simulink model "decentralized_closedloop"  (Simulink 7.4)
settings: Solver=ode45  StartTime=0.0  StopTime=400  FixedStep=0.05  MaxStep=0.05  RelTol=1e-3
values from neighbouring files (symbols this model uses):
  Ts = 0.05    [test_predictions.m]
  UWT = kron(eye(m),diag(UW'))    [test_predictions.m]
  xtotalsize = xsize + 2*sum(n_delay) + 2*dsize    [MpcSetup.m]
  yref = 0.2    [test_predictions.m]
  YWT = kron(eye(p),diag(YW'))    [test_predictions.m]
undefined symbols (not defined in the file or in its folder): n_controller_iterations, ucontrolsize, yss
libraries: lib_parallel_comp x1
settings Model: Creator=chkajon  LastModifiedBy=katie
settings SFSimCC: SimUserSources=../call_qpoases_m/call_qpoases.c
settings SFSimCC: SimUserIncludeDirs=|
  | ../call_qpoases_m/qpoases3/src
  | ../call_qpoases_m/qpoases3/include

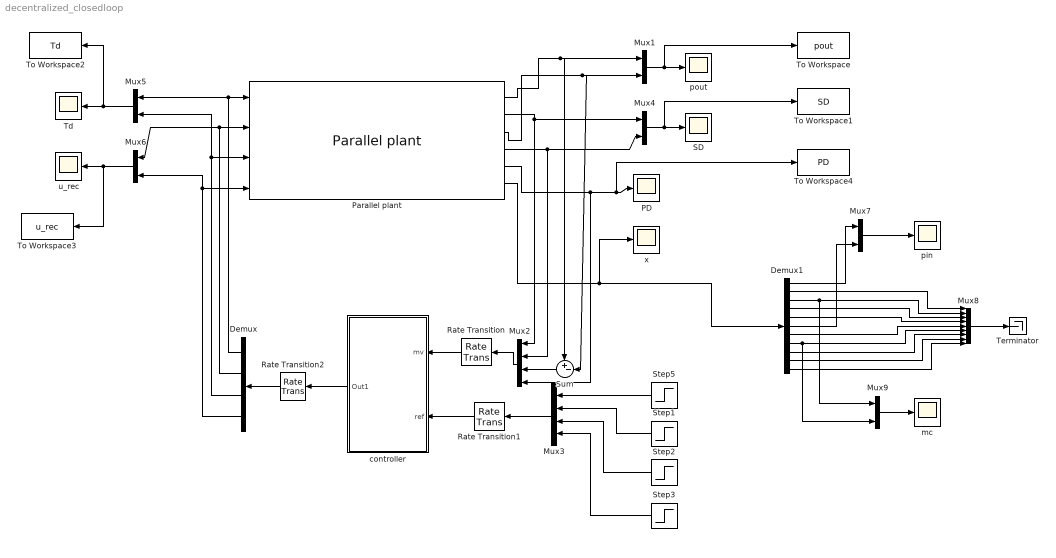
== system decentralized_closedloop ==
  Demux : Demux
  Demux1 : Demux  Outputs=11
  Mux{1,4..7,9} (6 alike) : Mux  Inputs=2
  Mux2 : Mux
  Mux3 : Mux
  Mux8 : Mux  Inputs=9
  PD : Scope
      settings: TimeRange=100  YMin=1.1  YMax=1.26  SaveName=SD1  DataFormat=Array
  Parallel plant : lib_parallel_comp/Parallel plant  SystemSampleTime=-1  disturbances_on=on  disturbances_symm=off  dist_t_in=tdist  dist1_in=udist1  dist2_in=udist2
  Rate Transition : RateTransition  X0=yss
  Rate Transition1 : RateTransition  X0=yref
  Rate Transition2 : RateTransition
  SD : Scope
      settings: TimeRange=100  YMin=-2.5  YMax=1.5  SaveName=SD3  DataFormat=Array
  Step1 : Step  Time=0  Before=0.22  After=0.22  SampleTime=0
  Step2 : Step  Time=0  After=0  SampleTime=0
  Step3 : Step  Time=0  Before=1.12  After=1.12  SampleTime=0
  Step5 : Step  Time=0  Before=0.22  After=0.22  SampleTime=0
  Sum : Sum  Inputs=+-|  OutDataType=fixdt(1, 16)  OutScaling=2^0
  Td : Scope
      settings: TimeRange=100  YMin=-0.15  YMax=0.25  SaveName=SD4  DataFormat=Array
  Terminator : Terminator
  To Workspace : ToWorkspace  VariableName=pout  SampleTime=-1  SaveFormat=Structure With Time
  To Workspace1 : ToWorkspace  VariableName=SD  SampleTime=-1  SaveFormat=Structure With Time
  To Workspace2 : ToWorkspace  VariableName=Td  SampleTime=-1  SaveFormat=Structure With Time
  To Workspace3 : ToWorkspace  VariableName=u_rec  SampleTime=-1  SaveFormat=Structure With Time
  To Workspace4 : ToWorkspace  VariableName=PD  SampleTime=-1  SaveFormat=Structure With Time
  controller : Subsystem  TreatAsAtomicUnit=on  SystemSampleTime=Ts
  mc : Scope
      settings: TimeRange=200  YMin=0.1175  YMax=0.155  SaveName=SD8  DataFormat=Array
  pin : Scope
      settings: TimeRange=200  YMin=0.89  YMax=1  SaveName=SD7  DataFormat=Array
  pout : Scope
      settings: TimeRange=100  YMin=1.38778e-017  YMax=0.4  SaveName=SD2  DataFormat=Array
  u_rec : Scope
      settings: TimeRange=100  YMin=-3.46945e-018  YMax=0.11  SaveName=SD5  DataFormat=Array
  x : Scope
      settings: TimeRange=85  YMin=1.1125  YMax=1.1141  SaveName=SD6  DataFormat=Array
  wires:
  controller/1(Out1) -> Rate Transition2/1
  Mux2/1 -> Rate Transition/1
  Mux3/1 -> Rate Transition1/1
  Rate Transition/1 -> controller/1(mv)
  Rate Transition1/1 -> controller/2(ref)
  Rate Transition2/1 -> Demux/1
  Demux/1 -> Mux5/1, Parallel plant/1
  Demux/2 -> Mux6/1, Parallel plant/2
  Demux/3 -> Mux5/2, Parallel plant/3
  Demux/4 -> Mux6/2, Parallel plant/4
  Step5/1 -> Mux3/1
  Step1/1 -> Mux3/2
  Step2/1 -> Mux3/3
  Step3/1 -> Mux3/4
  Parallel plant/1 -> Mux1/1, Sum/1
  Parallel plant/5 -> PD/1, To Workspace4/1, Mux2/4
  Parallel plant/2 -> Mux4/1, Mux2/1
  Parallel plant/3 -> Mux1/2, Sum/2
  Mux4/1 -> SD/1, To Workspace1/1
  Mux1/1 -> pout/1, To Workspace/1
  Mux5/1 -> Td/1, To Workspace2/1
  Mux6/1 -> u_rec/1, To Workspace3/1
  Parallel plant/6 -> x/1, Demux1/1
  Demux1/1 -> Mux7/1
  Demux1/6 -> Mux7/2
  Demux1/2 -> Mux8/1
  Demux1/3 -> Mux8/2, Mux9/1
  Demux1/4 -> Mux8/3
  Demux1/5 -> Mux8/4
  Demux1/7 -> Mux8/5
  Demux1/8 -> Mux8/6, Mux9/2
  Demux1/9 -> Mux8/7
  Demux1/10 -> Mux8/8
  Demux1/11 -> Mux8/9
  Mux8/1 -> Terminator/1
  Mux7/1 -> pin/1
  Mux9/1 -> mc/1
  Parallel plant/4 -> Mux4/2, Mux2/2
  Sum/1 -> Mux2/3

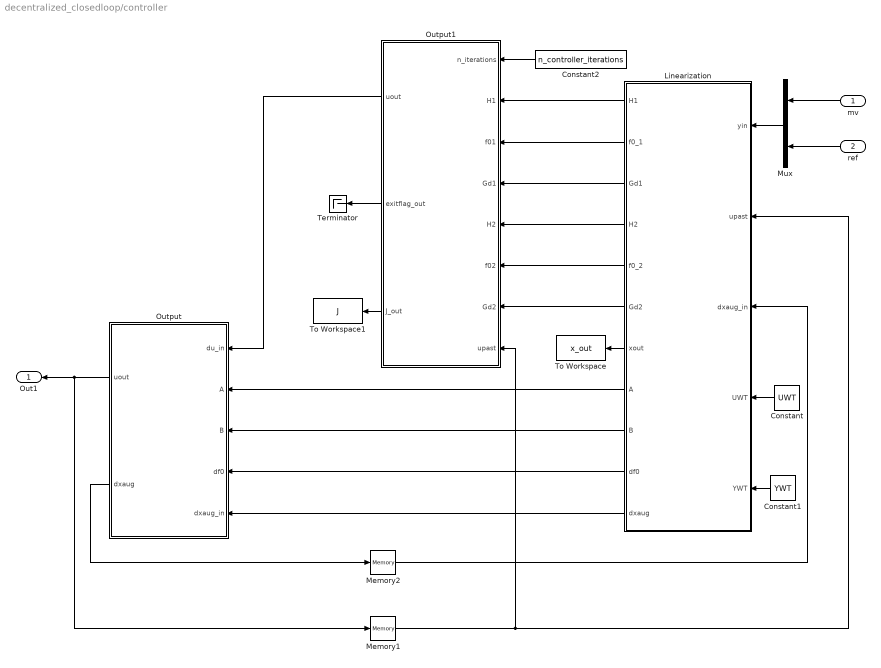
== system decentralized_closedloop/controller ==
  mv : Inport
  ref : Inport  Port=2
  Constant : Constant  Value=UWT  OutDataType=fixdt(1, 16)  OutScaling=2^0
  Constant1 : Constant  Value=YWT  OutDataType=fixdt(1, 16)  OutScaling=2^0
  Constant2 : Constant  Value=n_controller_iterations  OutDataType=fixdt(1, 16)  OutScaling=2^0
  Linearization : Stateflow chart  SystemSampleTime=Ts
  Memory1 : Memory  X0=zeros(2*ucontrolsize,1)  InheritSampleTime=on
  Memory2 : Memory  X0=zeros(xtotalsize,1)  InheritSampleTime=on
  Mux : Mux  Inputs=2
  Output : Stateflow chart  SystemSampleTime=Ts
  Output1 : Stateflow chart  SystemSampleTime=Ts
  Terminator : Terminator
  To Workspace : ToWorkspace  VariableName=x_out  SampleTime=-1  SaveFormat=Structure With Time
  To Workspace1 : ToWorkspace  VariableName=J  SampleTime=-1  SaveFormat=Structure
  Out1 : Outport
  wires:
  mv/1 -> Mux/1
  ref/1 -> Mux/2
  Memory1/1 -> Linearization/2(upast), Output1/8(upast)
  Memory2/1 -> Linearization/3(dxaug_in)
  Output/1(uout) -> Memory1/1, Out1/1
  Output/2(dxaug) -> Memory2/1
  Output1/1(uout) -> Output/1(du_in)
  Linearization/7(xout) -> To Workspace/1
  Linearization/8(A) -> Output/2(A)
  Linearization/9(B) -> Output/3(B)
  Linearization/10(df0) -> Output/4(df0)
  Linearization/11(dxaug) -> Output/5(dxaug_in)
  Linearization/1(H1) -> Output1/2(H1)
  Linearization/2(f0_1) -> Output1/3(f01)
  Linearization/3(Gd1) -> Output1/4(Gd1)
  Linearization/4(H2) -> Output1/5(H2)
  Linearization/5(f0_2) -> Output1/6(f02)
  Linearization/6(Gd2) -> Output1/7(Gd2)
  Mux/1 -> Linearization/1(yin)
  Constant/1 -> Linearization/4(UWT)
  Constant1/1 -> Linearization/5(YWT)
  Output1/2(exitflag_out) -> Terminator/1
  Output1/3(J_out) -> To Workspace1/1
  Constant2/1 -> Output1/1(n_iterations)

== matlab function controller/Output ==
  data: du_in input double; A input double; B input double; df0 input double; uout output double; dxaug_in input double; dxaug output double
function [uout,dxaug]  = fcn(du_in, A, B, df0, dxaug_in)
%#eml
persistent upast
eml.extrinsic('disp');
eml.extrinsic('toc');
eml.extrinsic('tic');
eml.extrinsic('num2str');
eml.extrinsic('keyboard');
eml.extrinsic('quadprog');



[~, ~, xsize, ~, ~] = const_sim();
[n_delay,~,ucontrolsize,~,m] = const_mpc();

if isempty(upast)
    tic
    upast = zeros(ucontrolsize*2,1);
    time = toc;
    disp(['Preparation time: ' num2str(time)]);
end

% take only the first move from du
du = [du_in(1:ucontrolsize,1); du_in(1+m*ucontrolsize:(m+1)*ucontrolsize,1)];

% Apply next input
u_new = upast + du;

% value of x about which we linearized
xlin = dxaug_in;
xlin(xsize+1:end) = 0;
xlin(xsize+1) = upast(2);
xlin(xsize+1+n_delay(2)) = upast(4);

dxaug = B*[u_new(1)-upast(1);u_new(2);u_new(3)-upast(3);u_new(4)] + A*(dxaug_in-xlin) + df0;

upast = u_new;
uout = u_new;

== matlab function controller/Linearization ==
  data: yin input double; H1 output double; f0_1 output double; Gd1 output double; H2 output double; f0_2 output double; Gd2 output double; xout output double; A output double; B output double; df0 output double; dxaug output double; upast input double; dxaug_in input double; UWT input double; YWT input double
function [H1, f0_1, Gd1, H2, f0_2, Gd2, xout, A, B, df0, dxaug]  = fcn(yin, upast, dxaug_in,UWT,YWT)
%#eml
% persistent C_new M LB UB Ga Gb Gc H Ain b A B upast xinit
persistent M xinit y_old C 
eml.extrinsic('disp');
eml.extrinsic('toc');
eml.extrinsic('tic');
eml.extrinsic('num2str');
eml.extrinsic('keyboard');
eml.extrinsic('quadprog');



[~, ~, xsize, ~, ysize] = const_sim();
% [n_delay,dsize,~,p] = const_mpc();

if isempty(M)
    tic
    [C,M,~,~,~,~,xinit] = get_constant_matrices();
%     y_old = zeros(ysize,1);
    y_old = [0.2175; 0.2175; 0; 1.12];
%     y_old = yss;
    time = toc;
    disp(['Preparation time: ' num2str(time)]);
end


y = yin(1:ysize);
yref = yin(ysize+1:end);

% Estimate state info
dxaug = dxaug_in + M*(y - y_old - C*(dxaug_in));

% Use state input info to calculate x, y
xinit(1:xsize) = xinit(1:xsize)+dxaug(1:xsize);
xinit(xsize+1:end) = dxaug(xsize+1:end);

xout = xinit;

% get matrices
[A,B,C,df0,H1,H2,f0_1,f0_2,Gd1,Gd2] = get_qp_matrices(xinit,upast,yref-y,UWT,YWT);

== matlab function controller/Output1 ==
  data: n_iterations input double; H1 input double; f01 input double; Gd1 input double; H2 input double; uout output double; f02 input double; exitflag_out output double; Gd2 input double; J_out output double; upast input double
function [uout,exitflag_out,J_out]  = fcn(n_iterations, H1, f01, Gd1, H2, f02, Gd2, upast)
%#eml
% persistent C_new M LB UB Ga Gb Gc H Ain b A B upast xinit
persistent LB UB Ain b usol_past
eml.extrinsic('disp');
eml.extrinsic('toc');
eml.extrinsic('tic');
eml.extrinsic('num2str');
eml.extrinsic('keyboard');

[~,~,usize,~,m] = const_mpc();


if isempty(LB)
    tic
    [~,~,UB,LB,b,Ain] = get_constant_matrices();
    usol_past = zeros(m*usize, 2);
    time = toc;
    disp(['Preparation time: ' num2str(time)]);
end

n_max_iterations = 3;

du_other1 = usol_past(:,1);
du_other2 = usol_past(:,2);

% Get reference and input vector
Upast1 = zeros(m*usize,1);
Upast2 = zeros(m*usize,1);
for i=1:m
    Upast1(1+(i-1)*usize:i*usize,1) = upast(1:usize);
    Upast2(1+(i-1)*usize:i*usize,1) = upast(usize+1:2*usize);
end

% Update bounds
LBa1 = LB - Upast1;
UBa1 = UB - Upast1;

LBa2 = LB - Upast2;
UBa2 = UB - Upast2;

J_out = zeros(n_max_iterations,2);

uout = zeros(2*m*usize,1);

exitflag_out = 0;


for i=1:n_max_iterations
    % Update linear term to add effect of other compressor
    f1 = f01 + du_other1'*Gd1;
    f2 = f02 + du_other2'*Gd2;
    
    % Solve QP
    lbA = -inf(size(Ain,1),1);
    [usol1,J1] = call_qpoases_m(H1,f1,Ain,LBa1,UBa1,lbA,b);
    [usol2,J2,exitflag] = call_qpoases_m(H2,f2,Ain,LBa2,UBa2,lbA,b);
    exitflag_out = exitflag(1,1);
    J_out(i,:) = [J1(1,1), J2(1,1)];
    
    for j=1:m*usize
        du_other1(j) = usol2(j);
        du_other2(j) = usol1(j);
    end
    
    
    if i==n_iterations
        % Output
        for j=1:m*usize
            uout(j) = usol1(j);
            uout(j+m*usize) = usol2(j);
        end
        if m>1
            for j=1:(m-1)*usize
                usol_past(j,:) = [usol1(usize+j), usol2(usize+j)];
            end
            usol_past((m-1)*usize+1:m*usize) = usol_past((m-2)*usize+1:(m-1)*usize);
        end
    end
end
